simulink model "hierarchical_controller"  (R2024b)
settings: Solver=VariableStepAuto  StartTime=0.0  StopTime=t(end)  RelTol=1e-3
InitFcn:
  | %% UAV PARAMETERS
  | m = 0.5;
  | Ib = diag([0.0023 0.0023 0.00509]);
  | 
  | %% SAMPLING TIME
  | Ts=0.001;
  | 
  | %% TRAJECTORY
  | 
  | % time
  | t = t_tot;
  | 
  | % initial position
  | p0x = points(1,1);
  | p0y = points(1,2);
  | p0z = - points(1,3); % ENU -> NED
  | p0 = [p0x p0y p0z];
  | 
  | % trajectory
  | csi_d=p; dot_csi_d=p_dot; ddot_csi_d=p_ddot;
  | psi_d=zeros(1,length(t)); dot_psi_d=zeros(1,length(t)); ddot_psi_d=zeros(1,length(t));
values from neighbouring files (symbols this model uses):
  p = [p segments(i:i+2,:)]    [main_trajectory.m]
  p_ddot = [p_ddot segments_ddot(i:i+2,:)]    [main_trajectory.m]
  p_dot = [p_dot segments_dot(i:i+2,:)]    [main_trajectory.m]
  points = zeros(n,3)    [casual_points.m]    (also in defined_points.m = [0 0 0.2)
  t_tot = [t_tot t_temp(i,:)]    [main_trajectory.m]
libraries: simulink x2, cstblocks x2, dspsigops x2, robotcorelib x1, uavutilslib x1
settings Model: Creator=ricca  LastModifiedBy=ricca

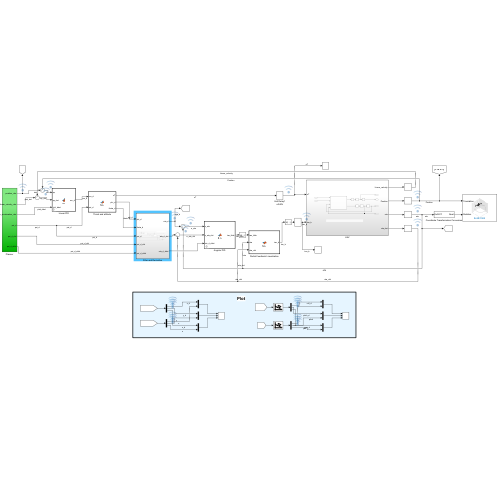
[thumbnail: Simulink's stored preview of the top-level diagram]
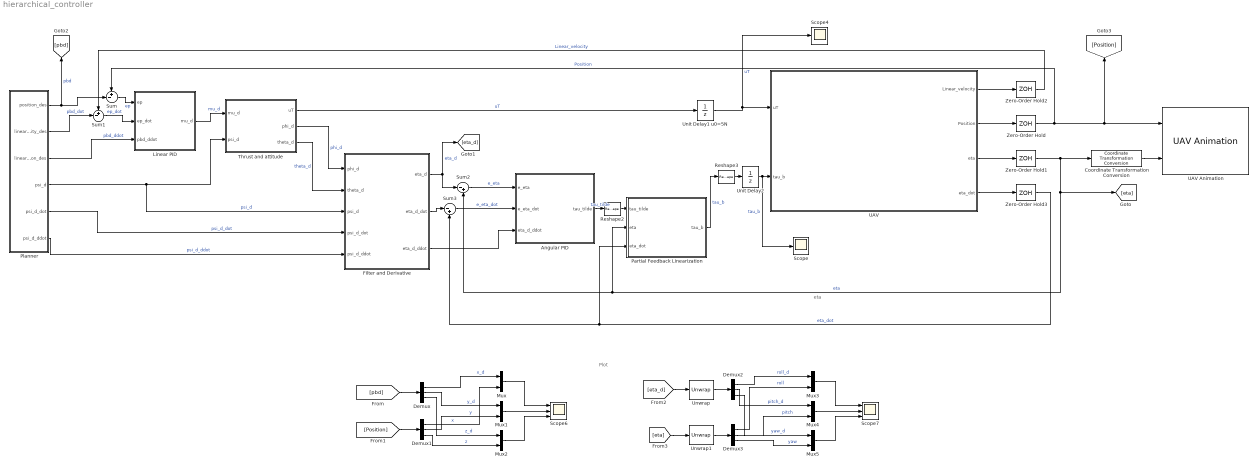
== system hierarchical_controller ==
  note: Plot
  note: eta
  Angular PID : MATLAB Function  TreatAsAtomicUnit=on  mask(Angular PID){Ke=[100*eye(3) 100*eye(3)]}
      mask help: Ke ∈ R^(3x6)
  Coordinate Transformation Conversion : robotcorelib/Coordinate Transformation Conversion  InputRepresentation=Euler Angles  InputEulerSequence=XYZ  ShowTrVecInputPort=on  OutputRepresentation=Quaternion  OutputEulerSequence=ZYX  ShowTrVecOutputPort=on  SimulateUsing=Interpreted execution
  Demux{,1..3} (4 alike) : Demux  Outputs=3
  Filter and Derivative : Subsystem
  Linear PID : MATLAB Function  TreatAsAtomicUnit=on  mask(Position PID){Kp=[100*eye(3) 10*eye(3)]}
      mask help: Kp ∈ R^(3x6)
  Mux{,1..5} (6 alike) : Mux  Inputs=2
  Partial Feedback Linearization : MATLAB Function  TreatAsAtomicUnit=on
  Planner : Subsystem
  Reshape2 : Reshape
  Reshape3 : Reshape
  Scope : Scope
  Scope4 : Scope
  Scope6 : Scope  NumInputPorts=3
  Scope7 : Scope  NumInputPorts=3
  Sum : Sum  Inputs=+-|
  Sum1 : Sum  Inputs=+-|
  Sum2 : Sum  Inputs=|-+
  Sum3 : Sum  Inputs=|-+
  Thrust and attitude : MATLAB Function  TreatAsAtomicUnit=on
  UAV : Subsystem
  UAV Animation : uavutilslib/UAV Animation  NumUAV=1  DynamicUAVConfig=off  UAVType=Multirotor  UAVSize=1  UAVColor=[1 0 0]  UAVTrajectoryAlpha=1  InertialZDirection=Down  RotationFormat=Quaternion  DrawMarkers=off  SampleTime=-1
  Unit Delay1 u0=5N : UnitDelay  InitialCondition=5  SampleTime=Ts
  Unit Delay2 : UnitDelay  InitialCondition=[0 0 0]  SampleTime=Ts
  Unwrap : dspsigops/Unwrap  tol=pi  InputProcessing=Columns as channels (frame based)  running=off
  Unwrap1 : dspsigops/Unwrap  tol=pi  InputProcessing=Columns as channels (frame based)  running=off
  Zero-Order Hold{,1..3} (4 alike) : ZeroOrderHold  SampleTime=-1
  wires:
  Zero-Order Hold1/1 -> Coordinate Transformation Conversion/1, Sum2/2, Partial Feedback Linearization/2(eta), [eta]  "eta"
  Coordinate Transformation Conversion/1 -> UAV Animation/2
  Thrust and attitude/1(uT) -> Unit Delay1 u0=5N/1  "uT"
  Partial Feedback Linearization/1(tau_b) -> Reshape3/1  "tau_b"
  Linear PID/1(mu_d) -> Thrust and attitude/1(mu_d)  "mu_d"
  Zero-Order Hold/1 -> Sum/1, UAV Animation/1, [Position]  "Position"
  Sum/1 -> Linear PID/1(ep)  "ep"
  Planner/1(position_des) -> Sum/2, [pbd]  "pbd"
  Zero-Order Hold2/1 -> Sum1/1  "Linear_velocity"
  Planner/2(linear_velocity_des) -> Sum1/2  "pbd_dot"
  Sum1/1 -> Linear PID/2(ep_dot)  "ep_dot"
  Planner/3(linear_acceleration_des) -> Linear PID/3(pbd_ddot)  "pbd_ddot"
  Planner/4(psi_d) -> Filter and Derivative/3(psi_d), Thrust and attitude/2(psi_d)  "psi_d"
  Angular PID/1(tau_tilde) -> Reshape2/1  "tau_tilde"
  Sum2/1 -> Angular PID/1(e_eta)  "e_eta"
  Zero-Order Hold3/1 -> Sum3/2, Partial Feedback Linearization/3(eta_dot)  "eta_dot"
  Sum3/1 -> Angular PID/2(e_eta_dot)  "e_eta_dot"
  Planner/5(psi_d_dot) -> Filter and Derivative/4(psi_d_dot)  "psi_d_dot"
  Planner/6(psi_d_ddot) -> Filter and Derivative/5(psi_d_ddot)  "psi_d_ddot"
  Thrust and attitude/2(phi_d) -> Filter and Derivative/1(phi_d)  "phi_d"
  Thrust and attitude/3(theta_d) -> Filter and Derivative/2(theta_d)  "theta_d"
  Filter and Derivative/2(eta_d_dot) -> Sum3/1
  Filter and Derivative/3(eta_d_ddot) -> Angular PID/3(eta_d_ddot)
  Reshape2/1 -> Partial Feedback Linearization/1(tau_tilde)
  Reshape3/1 -> Unit Delay2/1
  Unit Delay2/1 -> Scope/1, UAV/2(tau_b)  "tau_b"
  UAV/1(Linear_velocity) -> Zero-Order Hold2/1
  UAV/2(Position) -> Zero-Order Hold/1
  UAV/3(eta) -> Zero-Order Hold1/1
  UAV/4(eta_dot) -> Zero-Order Hold3/1
  Mux5/1 -> Scope7/3
  Demux1/2 -> Mux1/2  "y"
  [Position] -> Demux1/1
  Demux3/3 -> Mux5/2  "yaw"
  Mux4/1 -> Scope7/2
  [eta_d] -> Unwrap/1
  Demux3/1 -> Mux3/2  "roll"
  Demux/1 -> Mux/1  "x_d"
  Demux2/3 -> Mux5/1  "yaw_d"
  Demux/3 -> Mux2/1  "z_d"
  Demux1/1 -> Mux/2  "x"
  Unwrap/1 -> Demux2/1
  [eta] -> Unwrap1/1
  Mux1/1 -> Scope6/2
  [pbd] -> Demux/1
  Mux3/1 -> Scope7/1
  Mux/1 -> Scope6/1
  Unit Delay1 u0=5N/1 -> Scope4/1, UAV/1(uT)  "uT"
  Mux2/1 -> Scope6/3
  Demux2/2 -> Mux4/1  "pitch_d"
  Demux/2 -> Mux1/1  "y_d"
  Demux1/3 -> Mux2/2  "z"
  Unwrap1/1 -> Demux3/1
  Demux3/2 -> Mux4/2  "pitch"
  Demux2/1 -> Mux3/1  "roll_d"
  Filter and Derivative/1(eta_d) -> Sum2/1, [eta_d]  "eta_d"

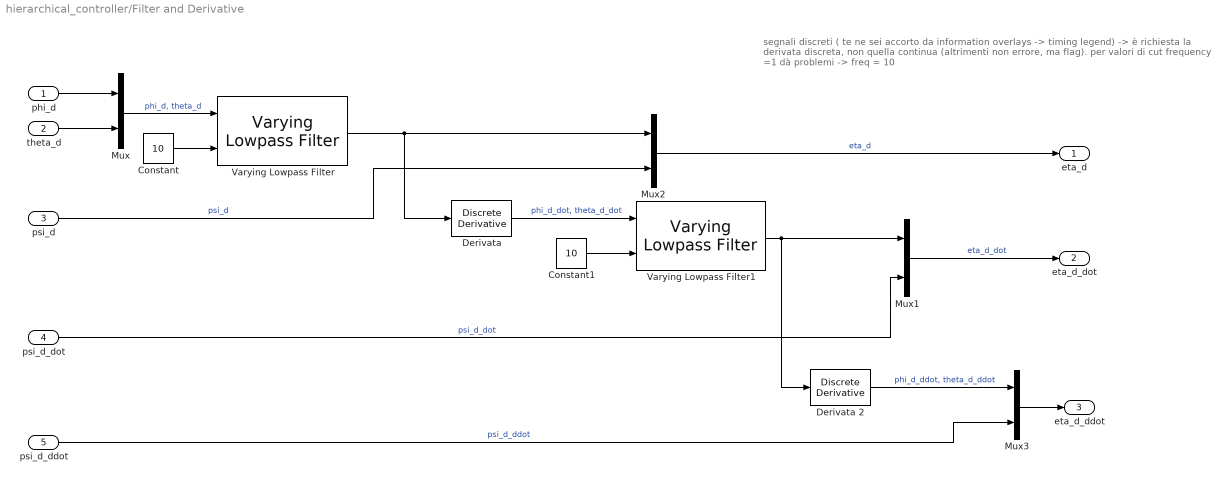
== system hierarchical_controller/Filter and Derivative ==
  note: segnali discreti ( te ne sei accorto da information overlays -> timing legend) -> è richiesta la derivata discreta, non quella continua (altrimenti non errore, ma flag).
      |
      | per valori di cut frequency =1 dà problemi -> freq = 10
  phi_d : Inport
  theta_d : Inport  Port=2
  psi_d : Inport  Port=3
  psi_d_dot : Inport  Port=4
  psi_d_ddot : Inport  Port=5
  Constant : Constant  Value=10
  Constant1 : Constant  Value=10
  Derivata : simulink/Discrete/Discrete Derivative  gainval=1.0  ICPrevScaledInput=0.0  OutMin=[]  OutMax=[]  OutDataType=fixdt(1, 16)  OutScaling=2^-10  DoSatur=off
  Derivata 2 : simulink/Discrete/Discrete Derivative  gainval=1.0  ICPrevScaledInput=0.0  OutMin=[]  OutMax=[]  OutDataType=fixdt(1, 16)  OutScaling=2^-10  DoSatur=off
  Mux{,1..3} (4 alike) : Mux  Inputs=2
  Varying Lowpass Filter : cstblocks/Linear Parameter Varying/Varying Lowpass Filter  N=1
  Varying Lowpass Filter1 : cstblocks/Linear Parameter Varying/Varying Lowpass Filter  N=1
  eta_d : Outport
  eta_d_dot : Outport  Port=2
  eta_d_ddot : Outport  Port=3
  wires:
  Derivata/1 -> Varying Lowpass Filter1/1  "phi_d_dot, theta_d_dot"
  theta_d/1 -> Mux/2
  phi_d/1 -> Mux/1
  psi_d/1 -> Mux2/2  "psi_d"
  Mux2/1 -> eta_d/1  "eta_d"
  psi_d_dot/1 -> Mux1/2  "psi_d_dot"
  Mux1/1 -> eta_d_dot/1  "eta_d_dot"
  Mux3/1 -> eta_d_ddot/1
  Derivata 2/1 -> Mux3/1  "phi_d_ddot, theta_d_ddot"
  psi_d_ddot/1 -> Mux3/2  "psi_d_ddot"
  Mux/1 -> Varying Lowpass Filter/1  "phi_d, theta_d"
  Varying Lowpass Filter/1 -> Derivata/1, Mux2/1
  Constant/1 -> Varying Lowpass Filter/2
  Varying Lowpass Filter1/1 -> Derivata 2/1, Mux1/1
  Constant1/1 -> Varying Lowpass Filter1/2

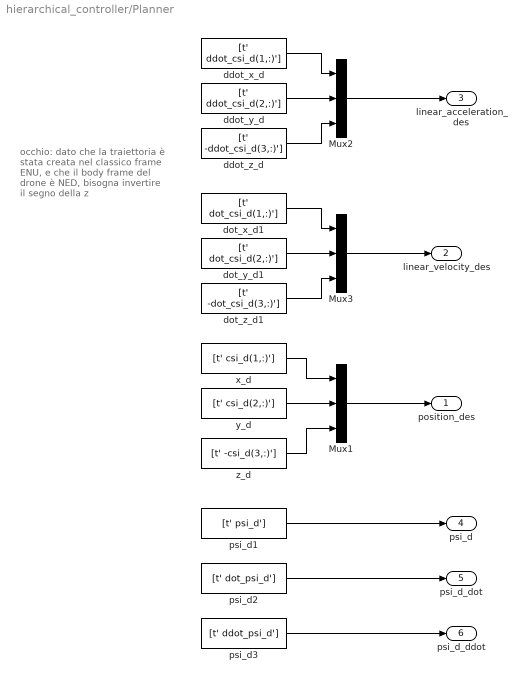
== system hierarchical_controller/Planner ==
  note: occhio: dato che la traiettoria è stata creata nel classico frame ENU, e che il body frame del drone è NED, bisogna invertire il segno della z
  Mux1 : Mux  Inputs=3
  Mux2 : Mux  Inputs=3
  Mux3 : Mux  Inputs=3
  ddot_x_d : FromWorkspace  VariableName=[t' ddot_csi_d(1,:)']  SampleTime=Ts
  ddot_y_d : FromWorkspace  VariableName=[t' ddot_csi_d(2,:)']  SampleTime=Ts
  ddot_z_d : FromWorkspace  VariableName=[t' -ddot_csi_d(3,:)']  SampleTime=Ts
  dot_x_d1 : FromWorkspace  VariableName=[t' dot_csi_d(1,:)']  SampleTime=Ts
  dot_y_d1 : FromWorkspace  VariableName=[t' dot_csi_d(2,:)']  SampleTime=Ts
  dot_z_d1 : FromWorkspace  VariableName=[t' -dot_csi_d(3,:)']  SampleTime=Ts
  psi_d1 : FromWorkspace  VariableName=[t' psi_d']  SampleTime=Ts
  psi_d2 : FromWorkspace  VariableName=[t' dot_psi_d']  SampleTime=Ts
  psi_d3 : FromWorkspace  VariableName=[t' ddot_psi_d']  SampleTime=Ts
  x_d : FromWorkspace  VariableName=[t' csi_d(1,:)']  SampleTime=Ts
  y_d : FromWorkspace  VariableName=[t' csi_d(2,:)']  SampleTime=Ts
  z_d : FromWorkspace  VariableName=[t' -csi_d(3,:)']  SampleTime=Ts
  position_des : Outport
  linear_velocity_des : Outport  Port=2
  linear_acceleration_des : Outport  Port=3
  psi_d : Outport  Port=4
  psi_d_dot : Outport  Port=5
  psi_d_ddot : Outport  Port=6
  wires:
  y_d/1 -> Mux1/2
  z_d/1 -> Mux1/3
  x_d/1 -> Mux1/1
  ddot_y_d/1 -> Mux2/2
  ddot_z_d/1 -> Mux2/3
  ddot_x_d/1 -> Mux2/1
  Mux2/1 -> linear_acceleration_des/1
  Mux1/1 -> position_des/1
  dot_y_d1/1 -> Mux3/2
  dot_z_d1/1 -> Mux3/3
  dot_x_d1/1 -> Mux3/1
  Mux3/1 -> linear_velocity_des/1
  psi_d1/1 -> psi_d/1
  psi_d2/1 -> psi_d_dot/1
  psi_d3/1 -> psi_d_ddot/1

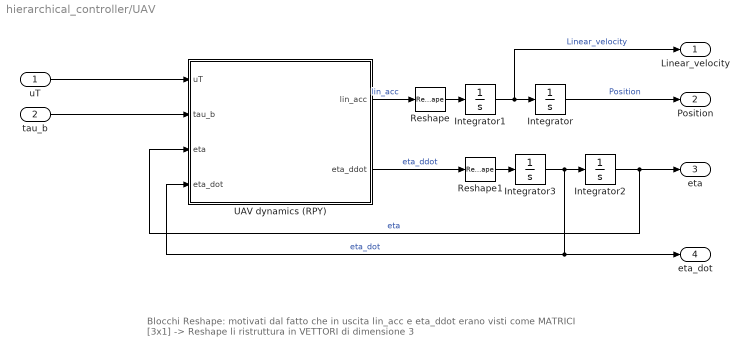
== system hierarchical_controller/UAV ==
  note: Blocchi Reshape: motivati dal fatto che in uscita lin_acc e eta_ddot erano visti come MATRICI [3x1] -> Reshape li ristruttura in VETTORI di dimensione 3
  uT : Inport
  tau_b : Inport  Port=2
  Integrator : Integrator  InitialCondition=p0
  Integrator1 : Integrator  InitialCondition=[0 0 0]
  Integrator2 : Integrator  InitialCondition=[0 0 0]
  Integrator3 : Integrator  InitialCondition=[0 0 0]
  Reshape : Reshape
  Reshape1 : Reshape
  UAV dynamics (RPY) : MATLAB Function  TreatAsAtomicUnit=on
  Linear_velocity : Outport
  Position : Outport  Port=2
  eta : Outport  Port=3
  eta_dot : Outport  Port=4
  wires:
  Integrator2/1 -> eta/1, UAV dynamics (RPY)/3(eta)  "eta"
  UAV dynamics (RPY)/1(lin_acc) -> Reshape/1  "lin_acc"
  Integrator1/1 -> Linear_velocity/1, Integrator/1  "Linear_velocity"
  Integrator3/1 -> eta_dot/1, UAV dynamics (RPY)/4(eta_dot), Integrator2/1  "eta_dot"
  Reshape1/1 -> Integrator3/1
  Reshape/1 -> Integrator1/1
  UAV dynamics (RPY)/2(eta_ddot) -> Reshape1/1  "eta_ddot"
  uT/1 -> UAV dynamics (RPY)/1(uT)
  tau_b/1 -> UAV dynamics (RPY)/2(tau_b)
  Integrator/1 -> Position/1  "Position"

== matlab function hierarchical_controller/Thrust and attitude ==
  data: mu_d input; uT output; phi_d output; theta_d output; psi_d input; m parameter
function [uT, phi_d, theta_d] = fcn(mu_d,psi_d,m)

uT = m*sqrt( mu_d(1)^2 + mu_d(2)^2 + (mu_d(3)-9.81)^2 );
phi_d = asin(m/uT*(mu_d(2)*cos(psi_d) - mu_d(1)*sin(psi_d)));
theta_d = atan((mu_d(1)*cos(psi_d) + mu_d(2)*sin(psi_d))/(mu_d(3)-9.81));

end

== matlab function hierarchical_controller/UAV/UAV dynamics (RPY) ==
  data: uT input; lin_acc output; tau_b input; eta input; eta_dot input; eta_ddot output; Ib parameter; m parameter
function [lin_acc, eta_ddot] = fcn(uT,tau_b, eta,eta_dot,Ib, m)

phi = eta(1);
theta = eta(2);
psi = eta(3);

phi_dot = eta_dot(1);
theta_dot = eta_dot(2);
psi_dot = eta_dot(3);

% Rb
Rb = [cos(theta)*cos(psi)    sin(phi)*sin(theta)*cos(psi) - cos(phi)*sin(psi)     cos(phi)*sin(theta)*cos(psi) + sin(phi)*sin(psi);
      cos(theta)*sin(psi)    sin(phi)*sin(theta)*sin(psi) + cos(phi)*cos(psi)     cos(phi)*sin(theta)*sin(psi) - sin(phi)*cos(psi);
          -sin(theta)                     sin(phi)*cos(theta)                                 cos(phi)*cos(theta)                ];

% Q(eta)
Q = [1          0       -sin(theta);
     0      cos(phi)     cos(theta)*sin(phi);
     0     -sin(phi)     cos(theta)*cos(phi)];

% Q_dot(eta)
Q_dot = [0        0                 cos(theta)*theta_dot;
         0    -sin(phi)*phi_dot    -sin(theta)*theta_dot*sin(phi) + cos(theta)*cos(phi)*phi_dot;
         0    -cos(phi)*phi_dot    -sin(theta)*theta_dot*cos(phi) - cos(theta)*sin(phi)*phi_dot];

% M(eta)
M = Q'*Ib*Q;

% C(eta,eta_dot)
C = Q'*skew(Q*eta_dot)*Ib*Q + Q'*Ib*Q_dot;


% RPY dynamic model 
lin_acc = 9.81*[0 0 1]'-(uT/m)*Rb*[0 0 1]';
eta_ddot = inv(M)*(-C*eta_dot + Q'*tau_b);

end


function S = skew(v)
if (numel(v)~= 1)
    S= [0 -v(3) v(2);
        v(3) 0 -v(1);
        -v(2) v(1) 0];
else
    S= zeros(3);
end
end

== matlab function hierarchical_controller/Linear PID ==
  data: ep input; mu_d output; ep_dot input; pbd_ddot input; Kp parameter
function mu_d = fcn(ep,ep_dot,pbd_ddot,Kp)

mu_d = -Kp*[ep;ep_dot] + pbd_ddot;

% acceleration handling
if mu_d(3) >= 9.81
    mu_d(3) = 9.8;
elseif mu_d(3) <= -9.81
    mu_d(3) = -9.8;
end


end

== matlab function hierarchical_controller/Partial Feedback Linearization ==
  data: tau_b output; tau_tilde input; eta input; eta_dot input; Ib parameter
function tau_b = fcn(tau_tilde,eta,eta_dot, Ib)

phi = eta(1);
theta = eta(2);
psi = eta(3);

phi_dot = eta_dot(1);
theta_dot = eta_dot(2);
psi_dot = eta_dot(3);


% Q(eta)
Q = [1          0       -sin(theta);
     0      cos(phi)     cos(theta)*sin(phi);
     0     -sin(phi)     cos(theta)*cos(phi)];

% Q_dot(eta)
Q_dot = [0        0                 cos(theta)*theta_dot;
         0    -sin(phi)*phi_dot    -sin(theta)*theta_dot*sin(phi) + cos(theta)*cos(phi)*phi_dot;
         0    -cos(phi)*phi_dot    -sin(theta)*theta_dot*cos(phi) - cos(theta)*sin(phi)*phi_dot];

% C(eta,eta_dot)
C = Q'*skew(Q*eta_dot)*Ib*Q + Q'*Ib*Q_dot;

% tau_b
tau_b = Ib*Q*tau_tilde  + inv(Q')*C*eta_dot;

end



function S = skew(v)
if (numel(v)~= 1)
    S= [0 -v(3) v(2);
        v(3) 0 -v(1);
        -v(2) v(1) 0];
else
    S= zeros(3);
end
end

== matlab function hierarchical_controller/Angular PID ==
  data: e_eta input; e_eta_dot input; eta_d_ddot input; tau_tilde output; Ke parameter
function tau_tilde = fcn(e_eta,e_eta_dot,eta_d_ddot,Ke)

tau_tilde = -Ke*[e_eta;e_eta_dot] + eta_d_ddot;

end
